simulink library "Sensors_Lib"  (Simulink 7.5)
settings: Solver=ode45  StartTime=0.0  StopTime=10.0  RelTol=1e-3
values from neighbouring files (symbols this model uses):
  AC = FASER_config    [UAV_config.m]    (also in UAV_modelconfig.mat = )
undefined symbols (not defined in the file or in its folder): SampleTime
libraries: Sensors_Lib x13, simulink x3
settings Model: Creator=austinmurch  LastModifiedBy=dept of AEM

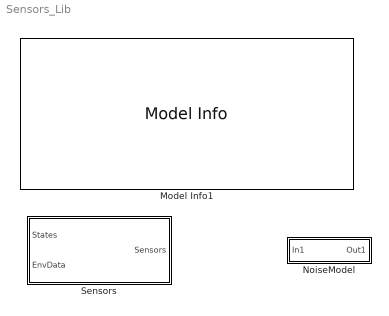
== system Sensors_Lib ==
  Model Info1 : simulink/Model-Wide Utilities/Model Info  SystemSampleTime=-1  InitialBlockCM=None  BlockCM=None  Frame=on  DisplayStringWithTags=|  HorizontalTextAlignment=Left  LeftAlignmentValue=0.02  SourceBlockDiagram=Sensors_Lib  TagMaxNumber=20
      | MODEL INFORMATION
      | Sensors Library
      | 
      | University of Minnesota
      | Aerospace Engineering and Mechanics
      | Copyright 2011 Regents of the University of Minnesota. All rights reserved.
      | 
      | == SVN Info ==
      | %<ModelVersion>
      | Last modified by %<LastModifiedBy> on %<LastModificationDate>
  NoiseModel : Subsystem  mask(Sensor Model){noise_on=1, sigma=AC.Sensors.IMU.p_noise, seed=878234, bias=0, scf=1, timestep=SampleTime}
      mask prompts: noise_on "on/off"; scf "scale factor:"
      mask help:
      | Add bias, scale factor, and white noise to a signal
      |
      | - 'on/off': 1 = noise on, 0 = noise off.
      | - 'sigma' : Standard deviation of white noise.
      | - 'seed'  : Random number seed.
      | - 'bias'  : Constant mean value offset of white noise.
      | - 'scale factor' : Scale factor applied to original signal.
      | - 'Timestep': Time step of the simulation
      mask Display: disp('bias/scf/noise')
  Sensors : Subsystem

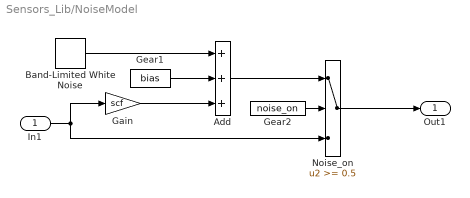
== system Sensors_Lib/NoiseModel ==
  In1 : Inport  OutDataType=sfix(16)  OutScaling=2^0
  Add : Sum  Inputs=+++  OutDataType=sfix(16)  OutScaling=2^-10
  Band-Limited White Noise : simulink/Sources/Band-Limited White Noise  SystemSampleTime=-1  Cov=sigma  Ts=timestep  seed=seed
  Gain : Gain  Gain=scf  ParameterDataType=sfix(16)  ParameterScaling=2^0  OutDataType=sfix(16)  OutScaling=2^0
  Gear1 : Constant  Value=bias  OutDataType=sfix(16)  OutScaling=2^0
  Gear2 : Constant  Value=noise_on  OutDataType=sfix(16)  OutScaling=2^0
  Noise_on : Switch  Threshold=0.5  SaturateOnIntegerOverflow=on  InputSameDT=on
  Out1 : Outport  OutDataType=sfix(16)  OutScaling=2^0
  wires:
  Noise_on/1 -> Out1/1
  Gear2/1 -> Noise_on/2
  Band-Limited White Noise/1 -> Add/1
  Add/1 -> Noise_on/1
  Gear1/1 -> Add/2
  Gain/1 -> Add/3
  In1/1 -> Noise_on/3, Gain/1

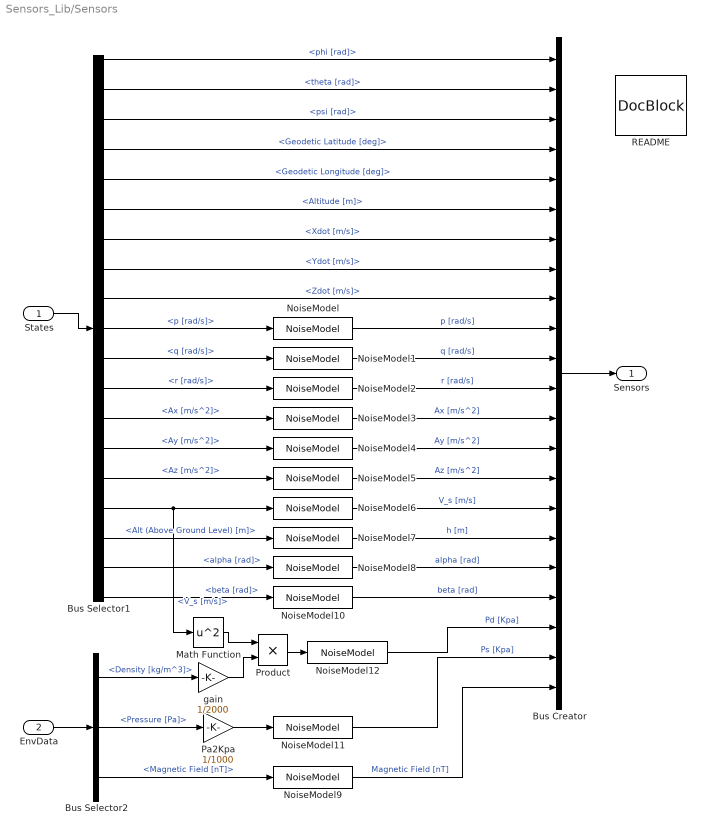
== system Sensors_Lib/Sensors ==
  States : Inport
  EnvData : Inport  Port=2
  Bus Creator : BusCreator  Inputs=22
  Bus Selector1 : BusSelector  OutputSignals=Euler [rad].phi [rad],Euler [rad].theta [rad],Euler [rad].psi [rad],Nav.Geodetic Latitude [deg],Nav.Geodetic Longitude [deg],Nav.Altitude [m],V_e [m/s].Xdot [m/s],V_e [m/s].Ydot [m/s],V_e [m/s].Zdot [m/s],AngVel [rad/s].p [rad/s],AngVel [rad/s].q [rad/s],AngVel [rad/s].r [rad/s],Accels [m/s^2].Ax [m/s^2],Accels [m/s^2].Ay [m/s^2],Accels [m/s^2].Az [m/s^2],WindAxesParam.V_s [m/s],Nav.Alt (Above Ground Level) [m],WindAxesParam.alpha [rad],WindAxesParam.beta [rad]
  Bus Selector2 : BusSelector  OutputSignals=Density [kg/m^3],Pressure [Pa],Magnetic Field [nT]
  Math Function : Math  Operator=square  OutDataType=fixdt(1, 16)  OutScaling=2^0  SaturateOnIntegerOverflow=on
  NoiseModel : Sensors_Lib/NoiseModel  SystemSampleTime=-1  noise_on=AC.Sensors.NoiseOn  sigma=AC.Sensors.IMU.p_noise  seed=878230  bias=AC.Sensors.IMU.p_bias  scf=AC.Sensors.IMU.p_scf  timestep=SampleTime
  NoiseModel1 : Sensors_Lib/NoiseModel  SystemSampleTime=-1  noise_on=AC.Sensors.NoiseOn  sigma=AC.Sensors.IMU.q_noise  seed=878231  bias=AC.Sensors.IMU.q_bias  scf=AC.Sensors.IMU.q_scf  timestep=SampleTime
  NoiseModel10 : Sensors_Lib/NoiseModel  SystemSampleTime=-1  noise_on=AC.Sensors.NoiseOn  sigma=AC.Sensors.AirData.beta_noise  seed=87828  bias=AC.Sensors.AirData.beta_bias  scf=AC.Sensors.AirData.beta_scf  timestep=SampleTime
  NoiseModel11 : Sensors_Lib/NoiseModel  SystemSampleTime=-1  noise_on=AC.Sensors.NoiseOn  sigma=AC.Sensors.AirData.Ps_noise  seed=8782378  bias=AC.Sensors.AirData.Ps_bias  scf=AC.Sensors.AirData.Ps_scf  timestep=SampleTime
  NoiseModel12 : Sensors_Lib/NoiseModel  SystemSampleTime=-1  noise_on=AC.Sensors.NoiseOn  sigma=AC.Sensors.AirData.Pd_noise  seed=87823  bias=AC.Sensors.AirData.Pd_bias  scf=AC.Sensors.AirData.Pd_scf  timestep=SampleTime
  NoiseModel2 : Sensors_Lib/NoiseModel  SystemSampleTime=-1  noise_on=AC.Sensors.NoiseOn  sigma=AC.Sensors.IMU.r_noise  seed=878232  bias=AC.Sensors.IMU.r_bias  scf=AC.Sensors.IMU.r_scf  timestep=SampleTime
  NoiseModel3 : Sensors_Lib/NoiseModel  SystemSampleTime=-1  noise_on=AC.Sensors.NoiseOn  sigma=AC.Sensors.IMU.ax_noise  seed=878233  bias=AC.Sensors.IMU.ax_bias  scf=AC.Sensors.IMU.ax_scf  timestep=SampleTime
  NoiseModel4 : Sensors_Lib/NoiseModel  SystemSampleTime=-1  noise_on=AC.Sensors.NoiseOn  sigma=AC.Sensors.IMU.ay_noise  seed=878234  bias=AC.Sensors.IMU.ay_bias  scf=AC.Sensors.IMU.ay_scf  timestep=SampleTime
  NoiseModel5 : Sensors_Lib/NoiseModel  SystemSampleTime=-1  noise_on=AC.Sensors.NoiseOn  sigma=AC.Sensors.IMU.az_noise  seed=878235  bias=AC.Sensors.IMU.az_bias  scf=AC.Sensors.IMU.az_scf  timestep=SampleTime
  NoiseModel6 : Sensors_Lib/NoiseModel  SystemSampleTime=-1  noise_on=AC.Sensors.NoiseOn  sigma=AC.Sensors.AirData.ias_noise  seed=878236  bias=AC.Sensors.AirData.ias_bias  scf=AC.Sensors.AirData.ias_scf  timestep=SampleTime
  NoiseModel7 : Sensors_Lib/NoiseModel  SystemSampleTime=-1  noise_on=AC.Sensors.NoiseOn  sigma=AC.Sensors.AirData.h_noise  seed=87828  bias=AC.Sensors.AirData.h_bias  scf=AC.Sensors.AirData.h_scf  timestep=SampleTime
  NoiseModel8 : Sensors_Lib/NoiseModel  SystemSampleTime=-1  noise_on=AC.Sensors.NoiseOn  sigma=AC.Sensors.AirData.alpha_noise  seed=87828  bias=AC.Sensors.AirData.alpha_bias  scf=AC.Sensors.AirData.alpha_scf  timestep=SampleTime
  NoiseModel9 : Sensors_Lib/NoiseModel  SystemSampleTime=-1  noise_on=AC.Sensors.NoiseOn  sigma=[AC.Sensors.IMU.hx_noise, AC.Sensors.IMU.hy_noise,AC.Sensors.IMU.hz_noise]  seed=878237  bias=[AC.Sensors.IMU.hx_bias, AC.Sensors.IMU.hy_bias, AC.Sensors.IMU.hz_bias]  scf=[AC.Sensors.IMU.hx_scf, AC.Sensors.IMU.hy_scf, AC.Sensors.IMU.hz_scf]  timestep=SampleTime
  Pa2Kpa : Gain  Gain=1/1000  ParameterDataType=fixdt(1, 16)  ParameterScaling=2^0  OutDataType=fixdt(1, 16)  OutScaling=2^0
  Product : Product  OutDataType=fixdt(1, 16)  OutScaling=2^0  RndMeth=Zero
  README : simulink/Model-Wide Utilities/DocBlock  SystemSampleTime=-1  DocumentType=Text
      content=|
      | Sensors
      |
      | This block implements sensor models on selected signals. A generic block
      | is used that applies a bias, scale factor, and band limited white noise to
      | a given signal. The parameters for each block are stored in the aircraft
      | configuration data structure (AC):
      |
      | >> AC.Sensors
      |
      | ans =
      |
      |     NoiseOn: 1
      |         IMU: [1x1 struct]
      |     AirData: [1x1 struct]
      |
      | Note the "NoiseOn" boolean flag- by setting this flag to zero, the sensor
      | model will be disabled.
      |
      | Currently, the bias and scale factor errors are not used; only white noise
      | is applied.
  gain : Gain  Gain=1/2000  ParameterDataType=fixdt(1, 16)  ParameterScaling=2^0  OutDataType=fixdt(1, 16)  OutScaling=2^0
  Sensors : Outport  OutDataType=fixdt(1, 16)  OutScaling=2^0
  wires:
  NoiseModel9/1 -> Bus Creator/22  "Magnetic Field [nT]"
  NoiseModel11/1 -> Bus Creator/21  "Ps [Kpa]"
  NoiseModel12/1 -> Bus Creator/20  "Pd [Kpa]"
  NoiseModel10/1 -> Bus Creator/19  "beta [rad]"
  NoiseModel8/1 -> Bus Creator/18  "alpha [rad]"
  NoiseModel7/1 -> Bus Creator/17  "h [m]"
  NoiseModel6/1 -> Bus Creator/16  "V_s [m/s]"
  NoiseModel5/1 -> Bus Creator/15  "Az [m/s^2]"
  NoiseModel4/1 -> Bus Creator/14  "Ay [m/s^2]"
  NoiseModel3/1 -> Bus Creator/13  "Ax [m/s^2]"
  NoiseModel2/1 -> Bus Creator/12  "r [rad/s]"
  NoiseModel1/1 -> Bus Creator/11  "q [rad/s]"
  NoiseModel/1 -> Bus Creator/10  "p [rad/s]"
  Bus Selector1/9 -> Bus Creator/9  "<Zdot [m/s]>"
  Bus Selector1/8 -> Bus Creator/8  "<Ydot [m/s]>"
  Bus Selector1/7 -> Bus Creator/7  "<Xdot [m/s]>"
  Bus Selector1/6 -> Bus Creator/6  "<Altitude [m]>"
  Bus Selector1/5 -> Bus Creator/5  "<Geodetic Longitude [deg]>"
  Bus Selector1/4 -> Bus Creator/4  "<Geodetic Latitude [deg]>"
  Bus Selector1/3 -> Bus Creator/3  "<psi [rad]>"
  Bus Selector1/2 -> Bus Creator/2  "<theta [rad]>"
  Bus Selector1/1 -> Bus Creator/1  "<phi [rad]>"
  Bus Creator/1 -> Sensors/1
  Product/1 -> NoiseModel12/1
  gain/1 -> Product/2
  Math Function/1 -> Product/1
  Bus Selector2/1 -> gain/1  "<Density [kg/m^3]>"
  Pa2Kpa/1 -> NoiseModel11/1
  Bus Selector2/2 -> Pa2Kpa/1  "<Pressure [Pa]>"
  Bus Selector1/19 -> NoiseModel10/1  "<beta [rad]>"
  Bus Selector1/18 -> NoiseModel8/1  "<alpha [rad]>"
  EnvData/1 -> Bus Selector2/1
  Bus Selector1/17 -> NoiseModel7/1  "<Alt (Above Ground Level) [m]>"
  Bus Selector2/3 -> NoiseModel9/1  "<Magnetic Field [nT]>"
  Bus Selector1/16 -> Math Function/1, NoiseModel6/1  "<V_s [m/s]>"
  States/1 -> Bus Selector1/1
  Bus Selector1/10 -> NoiseModel/1  "<p [rad/s]>"
  Bus Selector1/11 -> NoiseModel1/1  "<q [rad/s]>"
  Bus Selector1/12 -> NoiseModel2/1  "<r [rad/s]>"
  Bus Selector1/13 -> NoiseModel3/1  "<Ax [m/s^2]>"
  Bus Selector1/14 -> NoiseModel4/1  "<Ay [m/s^2]>"
  Bus Selector1/15 -> NoiseModel5/1  "<Az [m/s^2]>"
